simulink model "mpc_control_horizon"  (R2020b)
settings: Solver=ode4  StartTime=0.0  StopTime=t_sim  FixedStep=T  RelTol=1e-3
values from neighbouring files (symbols this model uses):
  A = [0 0 1 0; 0 0 0 1; 0 0 0 0; 0 0 0 0]    [main.m]
  B = [0 0; 0 0; 1 0; 0 1]    [main.m]
  C = [1 0 0 0; 0 1 0 0]    [main.m]
  mpc_design = mpc_mtx_fun(mpc_par)    [main.m]
  ref = [8; 10]    [main.m]
  T = 0.01    [main.m]
  x0 = [2; 1; 0; 0]    [main.m]
undefined symbols (not defined in the file or in its folder): Ad_sys, Bd_sys, mpc_par
settings Model: Creator=vince  LastModifiedBy=vince
settings DataIOCC: ReturnWorkspaceOutputs=off
settings DebuggingCC: ReadBeforeWriteMsg=DisableAll  WriteAfterWriteMsg=DisableAll  WriteAfterReadMsg=DisableAll  MultiTaskDSMMsg=none
settings ModelReferenceCC: UpdateModelReferenceTargets=IfOutOfDate
settings SFSimCC: SFSimEcho=off

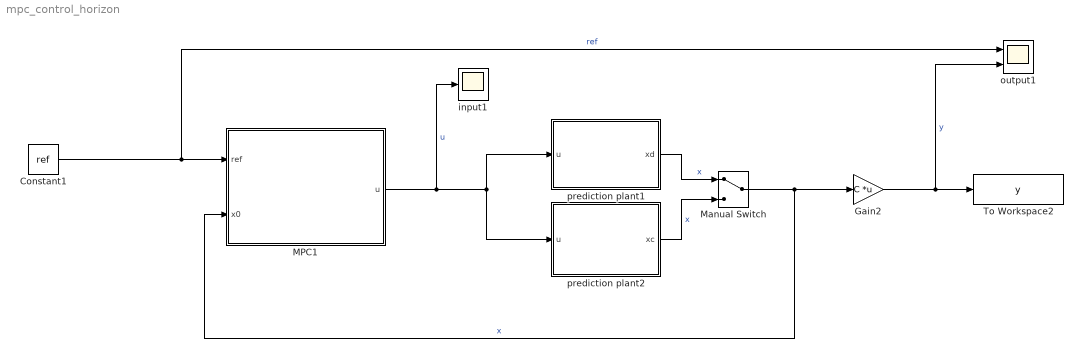
== system mpc_control_horizon ==
  Constant1 : Constant  Value=ref  SampleTime=-1
  Gain2 : Gain  Gain=C  Multiplication=Matrix(K*u) (u vector)
  MPC1 : Subsystem
  Manual Switch : ManualSwitch
  To Workspace2 : ToWorkspace  VariableName=y  SaveFormat=Timeseries  SampleTime=-1
  input1 : Scope
  output1 : Scope  NumInputPorts=2
  prediction plant1 : Subsystem
  prediction plant2 : Subsystem
  wires:
  Gain2/1 -> output1/2, To Workspace2/1  "y"
  Constant1/1 -> output1/1, MPC1/1(ref)  "ref"
  Manual Switch/1 -> MPC1/2(x0), Gain2/1  "x"
  prediction plant1/1(xd) -> Manual Switch/1  "x"
  MPC1/1(u) -> prediction plant1/1(u), prediction plant2/1(u), input1/1  "u"
  prediction plant2/1(xc) -> Manual Switch/2  "x"

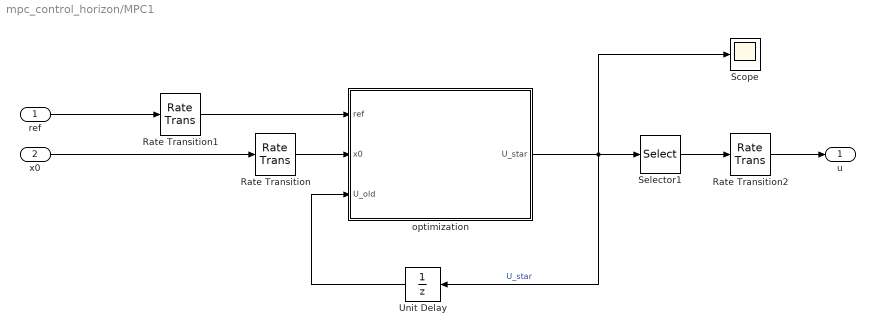
== system mpc_control_horizon/MPC1 ==
  ref : Inport
  x0 : Inport  Port=2
  Rate Transition : RateTransition  OutPortSampleTime=mpc_par.Ts
  Rate Transition1 : RateTransition  OutPortSampleTime=mpc_par.Ts
  Rate Transition2 : RateTransition  OutPortSampleTime=T
  Scope : Scope
  Selector1 : Selector  InputPortWidth=mpc_par.q*mpc_par.Nc  IndexOptions=Index vector (dialog)  Indices=1:mpc_par.q  OutputSizes=1
  Unit Delay : UnitDelay  InitialCondition=mpc_design.U0  SampleTime=mpc_par.Ts  HasFrameUpgradeWarning=on
  optimization : MATLAB Function  TreatAsAtomicUnit=on
  u : Outport
  wires:
  ref/1 -> Rate Transition1/1
  Unit Delay/1 -> optimization/3(U_old)
  Rate Transition/1 -> optimization/2(x0)
  optimization/1(U_star) -> Scope/1, Selector1/1, Unit Delay/1  "U_star"
  Rate Transition1/1 -> optimization/1(ref)
  Selector1/1 -> Rate Transition2/1
  x0/1 -> Rate Transition/1
  Rate Transition2/1 -> u/1

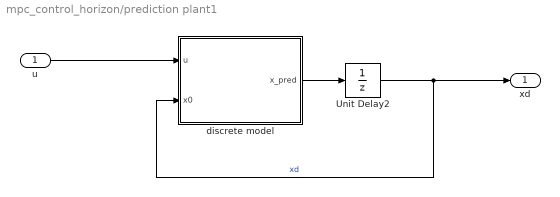
== system mpc_control_horizon/prediction plant1 ==
  u : Inport
  Unit Delay2 : UnitDelay  InitialCondition=x0  SampleTime=T  HasFrameUpgradeWarning=on
  discrete model : MATLAB Function  TreatAsAtomicUnit=on
  xd : Outport
  wires:
  discrete model/1(x_pred) -> Unit Delay2/1
  Unit Delay2/1 -> discrete model/2(x0), xd/1  "xd"
  u/1 -> discrete model/1(u)

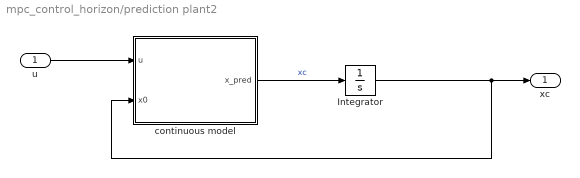
== system mpc_control_horizon/prediction plant2 ==
  u : Inport
  Integrator : Integrator  InitialCondition=x0
  continuous model : MATLAB Function  TreatAsAtomicUnit=on
  xc : Outport
  wires:
  u/1 -> continuous model/1(u)
  Integrator/1 -> xc/1, continuous model/2(x0)
  continuous model/1(x_pred) -> Integrator/1  "xc"

== matlab function mpc_control_horizon/prediction plant2/continuous model ==
  data: u input; x_pred output; x0 input; A parameter; B parameter
function x_pred = mpc_pred_cont(u, x0, A, B)

x = x0;
x_pred = A*x + B*u;

== matlab function mpc_control_horizon/MPC1/optimization ==
  data: ref input; U_star output; x0 input; U_old input; mpc_par parameter; mpc_design parameter
function U_star = mpc_optimization(ref, x0, U_old, mpc_par, mpc_design)
%% Documentation
%{
    INCOME: ref, x, U_old
    OUTCOME: U*, X_hat
%}


%% Assignment
n = mpc_par.n;
p = mpc_par.p;
q = mpc_par.q;
Np = mpc_par.Np;
Nc = mpc_par.Nc;


%% Reference
REF = repmat(ref, Np, 1);


%% Constraints
X_min = mpc_design.X_c(:,1);
X_max = mpc_design.X_c(:,2);
U_min = mpc_design.U_c(:,1);
U_max = mpc_design.U_c(:,2);
dU_min = mpc_design.dU_c(:,1);
dU_max = mpc_design.dU_c(:,2);


A_ineq = [-mpc_design.B_bar; mpc_design.B_bar;
        -eye(q*Nc); eye(q*Nc); 
        -eye(q*Nc); eye(q*Nc)];
b_ineq = [-X_min+mpc_design.A_bar*x0; X_max-mpc_design.A_bar*x0;
        -U_min; U_max;
        -dU_min-U_old; dU_max+U_old];

    
%% Objective function

H = mpc_design.R_bar + mpc_design.D_bar'*mpc_design.Q_bar*mpc_design.D_bar;
H = (H+H')/2;
f = (mpc_design.C_bar*x0-REF)'*mpc_design.Q_bar*(mpc_design.D_bar);


%% Optimization: J(u(k)) = U(k)'*H*U(k) + f'*U(k)

coder.extrinsic('quadprog');
% options = optimoptions('quadprog', 'Algorithm', 'active-set', 'Display', 'iter');

U_star = zeros(q*Nc, 1);
U_star = quadprog(H, f, A_ineq, b_ineq, [], [], [], [], []);

== matlab function mpc_control_horizon/prediction plant1/discrete model ==
  data: u input; x_pred output; x0 input; Ad_sys parameter; Bd_sys parameter
function x_pred = mpc_pred_disc(u, x0, Ad_sys, Bd_sys)

x = x0;
x_pred = Ad_sys*x + Bd_sys*u;
